simulink model "TestingModel"  (R2023b)
settings: Solver=VariableStepAuto  StartTime=0.0  StopTime=3.5  RelTol=1e-3
InitFcn:
  | run('Parameter_2M_DFIG_RSC.m')
values from neighbouring files (symbols this model uses):
  D = 0    [DefaultSimscapeValues.m]    (also in Newabccoordparam.m = 0.001)
  f = 60    [DefaultSimscapeValues.m]    (also in Newabccoordparam.m = 50)
  Fs = Vs*sqrt(2/3)/(2*pi*f)    [DefaultSimscapeValues.m]    (also in Newabccoordparam.m)
  fsw = 4e3    (= 4000)    [Newabccoordparam.m]
  J = 1.662    [DefaultSimscapeValues.m]    (also in Newabccoordparam.m = 127)
  ki_id = (wni^2)*Lr*sigma    (= 491.599501999)    [Newabccoordparam.m]
  ki_iq = ki_id    (= 491.599501999)    [Newabccoordparam.m]
  ki_n = ((wnn^2)*J)/p    (= 25400)    [Newabccoordparam.m]
  kp_id = (2*wni*sigma*Lr)-Rr    (= 0.5771)    [Newabccoordparam.m]
  kp_iq = kp_id    (= 0.5771)    [Newabccoordparam.m]
  kp_n = (2*wnn*J)/p    (= 2540)    [Newabccoordparam.m]
  Lm = 13.08/377    (= 0.0346949602122)    [DefaultSimscapeValues.m]    (also in Newabccoordparam.m = 0.0025)
  Lr = Lm + Lsi    (= 0.0354960212202)    [DefaultSimscapeValues.m]    (also in Newabccoordparam.m = 0.002587)
  Ls = Lm + Lsi    (= 0.0354960212202)    [DefaultSimscapeValues.m]    (also in Newabccoordparam.m = 0.002587)
  Lsi = 0.302/377    (= 0.000801061007958)    [DefaultSimscapeValues.m]    (also in Newabccoordparam.m = 8.7e-05)
  p = 2    [DefaultSimscapeValues.m]    (also in Newabccoordparam.m)
  Ps = 37300    [DefaultSimscapeValues.m]    (also in Newabccoordparam.m = 2000000)
  Rr = 0.228    [DefaultSimscapeValues.m]    (also in Newabccoordparam.m = 0.0029)
  Rs = 0.087    [DefaultSimscapeValues.m]    (also in Newabccoordparam.m = 0.0026)
  sigma = 1- Lm^2/(Ls*Lr)    (= 0.0446259584738)    [DefaultSimscapeValues.m]    (also in Newabccoordparam.m = 0.0661284179513)
  Tem = 12732    [Newabccoordparam.m]
  Vbus = Vr_stator*sqrt(2)    [Newabccoordparam.m]
  Vs = 460    [DefaultSimscapeValues.m]    (also in Newabccoordparam.m = 690)
undefined symbols (not defined in the file or in its folder): DiscIntNeverNeededParam
libraries: spsabctodq0Lib x3, eeGeneralControl x2, spsThreePhaseVIMeasurementLib x2, spsdq0toabcLib x2, spsAsynchronousMachineSIUnitsLib x1, spsDCVoltageSourceLib x1, spsGroundLib x1, spsPWMGenerator2LevelLib x1, spsThreePhaseProgrammableVoltageSourceLib x1, spsUniversalBridgeLib x1, sps_lib x1
settings Model: Creator=collins  LastModifiedBy=collins

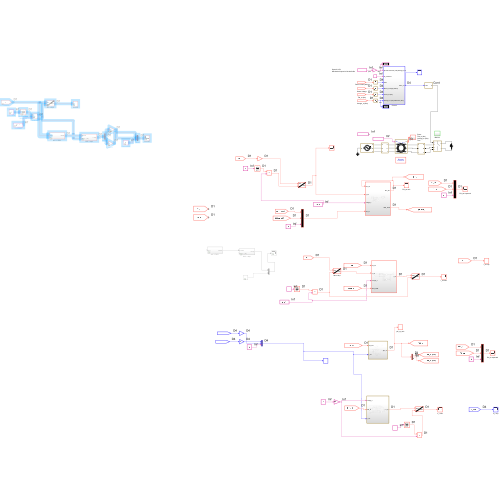
[thumbnail: Simulink's stored preview of the top-level diagram]
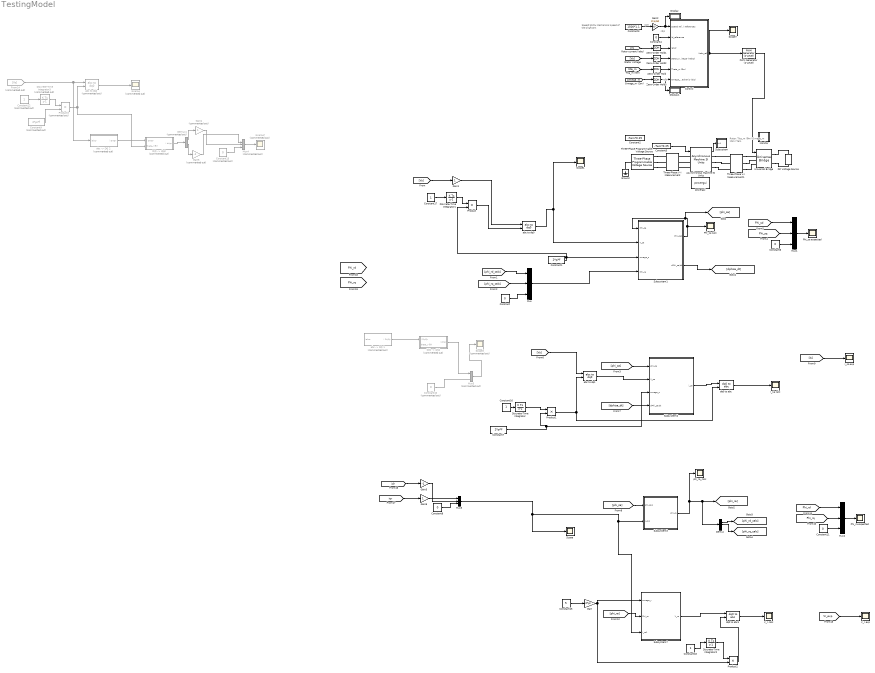
== system TestingModel ==
  note: rpm
  note: Rotor:
      | Tita_m (θm)
      | Omega_m (Ωm)
      | Tem
  note: rd/s
  note: rd/s
  note: Speed*110%
      | Mechanical speed of the shaft Ωm
  Asynchronous Machine SI Units : spsAsynchronousMachineSIUnitsLib/Asynchronous Machine SI Units  RotorType=Wound  PresetModel=No  MechanicalLoad=Torque Tm  ShowDetailedParameters=on  ReferenceFrame=Synchronous  Units=SI  MeasurementBus=off  NominalParameters=[ Ps Vs f ]  VoltageRatio=1  Stator=[ Rs , Lsi]  Rotor=[ Rr , Lsi]  Cage1=[ 0.022 0.226/377]  Cage2=[ 0.022 0.226/377]  Lm=Lm  Mechanical=[ J D 2 ]  PolePairs=2  InitialConditions=[1 0 0 0 0 0 0 0]  SimulateSaturation=off  Saturation=[14.03593122, 27.81365428, 53.79336849, 72.68890987, 97.98006896, 148.6815601, 215.7428561, 302.9841135, 420.4778367 ; 230, 322, 414, 460, 506, 552, 598, 644, 690]  LoadFlowParameters=1492000  TsPowergui=0  TsBlock=-1  IterativeModel=Trapezoidal non iterative  IterativeDiscreteModel=Trapezoidal non iterative  Pmec=0
      settings: AttributesFormatString=\n
  Constant{,4,6,8,11} (5 alike) : Constant  Value=0
  Constant1 : Constant  Value=2*pi*f
  Constant10 : Constant  Commented=on  Value=0
  Constant12 : Constant  Commented=on
  Constant13 : Constant  Commented=on  Value=0
  Constant15 : Constant  Value=5
  Constant16 : Constant
  Constant17 : Constant
  Constant18 : Constant
  Constant2 : Constant  Value=-Tem*0.25
  Constant3 : Constant  Value=1500*1.1
  Constant5 : Constant  Value=-Tem*0.25
  Constant7 : Constant  Value=2*pi*f
  Constant9 : Constant  Commented=on  Value=2*pi*f
  Control : Subsystem
  "D/Q -> d/q1" : Subsystem  Commented=on
  "D/Q -> d/q2" : Subsystem  Commented=on
  DC Voltage Source : spsDCVoltageSourceLib/DC Voltage Source  Amplitude=Vbus  Measurements=None
  Demux : Demux  Outputs=3
  Demux1 : Demux  Commented=on  Outputs=2
  Discrete-Time Integrator : DiscreteIntegrator  SampleTime=-1  ICPrevOutput=DiscIntNeverNeededParam  ICPrevScaledInput=DiscIntNeverNeededParam
  Discrete-Time Integrator1 : DiscreteIntegrator  SampleTime=-1  ICPrevOutput=DiscIntNeverNeededParam  ICPrevScaledInput=DiscIntNeverNeededParam
  Discrete-Time Integrator2 : DiscreteIntegrator  SampleTime=-1  ICPrevOutput=DiscIntNeverNeededParam  ICPrevScaledInput=DiscIntNeverNeededParam
  Discrete-Time Integrator3 : DiscreteIntegrator  Commented=on  SampleTime=-1  ICPrevOutput=DiscIntNeverNeededParam  ICPrevScaledInput=DiscIntNeverNeededParam
  Display : Display
  Display1 : Display
  From14 : From  Commented=on  GotoTag=Vs  TagVisibility=global
  Gain : Gain  Gain=2*pi
  Gain1 : Gain
  Gain2 : Gain  Gain=2*pi/60
  Gain3 : Gain  Gain=-1
  Gain4 : Gain  Commented=on
  Gain5 : Gain  Commented=on  Gain=-1
  Gain6 : Gain
  Ground : spsGroundLib/Ground  LConnTagsString=a
  Monitor : Subsystem
  Mux{,1..3} (4 alike) : Mux  Inputs=3
  Mux4 : Mux  Commented=on  Inputs=3
  Mux5 : Mux  Commented=on  Inputs=2
  PWM Generator (2-Level) : spsPWMGenerator2LevelLib/PWM Generator (2-Level)  ModulatorType=Three-phase bridge (6 pulses)  ModulatorMode=Unsynchronized  Fc=fsw  Pc=90  nF=27  MinMax="[ -1  1 ]"  SamplingTechnique=Natural  ModulatingSignals=off  m=0.8  Freq=60  Phase=0  Ts=0  ShowCarrierOutport=off
  Phi_ra expected : Scope
  Phi_sa calc : Scope
  Phi_sa expected : Scope
  Product : Product
  Product1 : Product
  Product2 : Product
  Product3 : Product  Commented=on
  Scope : Scope
  Scope1 : Scope
  Scope3 : Scope  Commented=on
  Scope7 : Scope
  Subsystem : Subsystem
  Subsystem1 : Subsystem
  Subsystem2 : Subsystem
  Subsystem3 : Subsystem
  Subsystem7 : Subsystem
  Three-Phase Programmable Voltage Source : spsThreePhaseProgrammableVoltageSourceLib/Three-Phase Programmable Voltage Source  PositiveSequence="[Vs  0 f]"  VariationEntity=None  VariationType=Table of time-amplitude pairs  VariationTypeAlt=Step  VariationStep=0.5  VariationRate=10  VariationMagnitude=0.3  VariationFrequency=2  VariationTiming=[1 2]  VariationPhaseA=off  Amplitudes=[1 0.8 1.2 1.0]  TimeValues=[0 0.1 0.15 0.2]  HarmonicGeneration=off  HarmonicA=[3 0.2 -25 0]  HarmonicB=[2 0.15 35 2]  Timing="[0.05  3]"  BusType=swing  Pref=0  Qref=0  Qmin=-inf  Qmax=inf
  Three-Phase V-I Measurement : spsThreePhaseVIMeasurementLib/Three-Phase V-I Measurement  VoltageMeasurement=phase-to-ground  SetLabelV=on  LabelV=Vs  Vpu=off  VpuLL=off  CurrentMeasurement=yes  SetLabelI=on  LabelI=Is  Ipu=off  Pbase=100e6  Vbase=500e3  OutputType=Complex  PhasorSimulation=off  PSBequivalent=0
  Three-Phase V-I Measurement1 : spsThreePhaseVIMeasurementLib/Three-Phase V-I Measurement  VoltageMeasurement=phase-to-phase  SetLabelV=on  LabelV=Vr  Vpu=off  VpuLL=off  CurrentMeasurement=yes  SetLabelI=on  LabelI=Ir  Ipu=off  Pbase=100e6  Vbase=500e3  OutputType=Complex  PhasorSimulation=off  PSBequivalent=0
  Universal Bridge : spsUniversalBridgeLib/Universal Bridge  Arms=3  SnubberResistance=1e5  SnubberCapacitance=inf  Device=Ideal Switches  Ron=1e-3  Lon=0  ForwardVoltages="[  0  0  ]"  ForwardVoltage=0  GTOparameters=[ 10e-6 , 20e-6 ]  IGBTparameters=[ 1e-6 , 2e-6 ]  Measurements=None  Measurements_2=None  converterType=Rectifier
  V_r calc : Scope
  V_r exp : Scope
  Zero-Order Hold{,1..3} (4 alike) : ZeroOrderHold  SampleTime=1/fsw
  "abc -> DQ 1" : Subsystem  Commented=on
  "abc -> DQ 2" : Subsystem  Commented=on
  abc to dq0 : spsabctodq0Lib/abc to dq0  Alignment=90 degrees behind phase A axis
  abc to dq1 : spsabctodq0Lib/abc to dq0  Alignment=90 degrees behind phase A axis
  abc to dq2 : spsabctodq0Lib/abc to dq0  Commented=on  Alignment=90 degrees behind phase A axis
  dq0 to abc : spsdq0toabcLib/dq0 to abc  Alignment=90 degrees behind phase A axis
  dq0 to abc1 : spsdq0toabcLib/dq0 to abc  Alignment=Aligned with phase A axis
  i_sa calc : Scope
  i_sa exp : Scope
  issame : Scope  Commented=on
  issame? : Scope  Commented=on
  phi_ra_calc : Scope
  powergui : sps_lib/powergui  Priority=1  SimulationMode=Discrete  SampleTime=15e-6  frequency=60  Iterations=50  frequencyindice=50  Pbase=100e6  ErrMax=1e-4  UnitsV=kV  UnitsW=MW  buscounter=0  FunctionMessages=off  echomessages=off  EnableUseOfTLC=off  CurrentSourceSwitches=off  DisableSnubberDevices=off  DisableRonSwitches=off  DisableVfSwitches=off  DisplayEquations=off  AutomaticDiscreteSolvers=off  SolverType=Tustin  Interpol=off  ExternalGateDelay=off  methode=off  Ts=0  x0status=blocks  SPID=off  SwTol=0  HookPort=off  NonlinearTolerance=1e-4  nMaxIteration=100  ContinueOnMaxIteration=off  RestoreLinks=warning  ResistiveCurrentMeasurement=off  Frange=[0:2:500]  Ylog=off  Xlog=on  ShowGrid=off  save=off  variable=ZData  structure=0  ZoomFFT=off  StartTime=0.0  cycles=1  DisplayStyle=1  fundamental=60  FreqAxis=off  MaxFrequency=1000  frequencyindicesteady=1  RmsSteady=1  display=off
  wires:
  Zero-Order Hold1/1 -> Control/3(iabcr)
  [Ir] -> Zero-Order Hold1/1
  [Vs] -> Zero-Order Hold2/1
  [omega_m] -> Zero-Order Hold3/1
  Zero-Order Hold2/1 -> Control/4(Stator_Voltage (Vabcs))
  Constant3/1 -> Gain2/1
  Zero-Order Hold/1 -> Control/5(Theta_m (θm))
  Constant4/1 -> Control/2(id_reference)
  Constant5/1 -> Asynchronous Machine SI Units/1
  PWM Generator (2-Level)/1 -> Universal Bridge/1
  Asynchronous Machine SI Units/1 -> Subsystem/1(In1)
  Zero-Order Hold3/1 -> Display1/1, Control/6(Omega_m (Ωm) Mechanic (rd/s))
  Gain2/1 -> Display/1, Control/1(Speed reference (rd/s) Omega_m (Ωm) references)
  [tita_m] -> Zero-Order Hold/1
  Control/1(Vabc_ref) -> Scope7/1, PWM Generator (2-Level)/1
  Subsystem1/1(Phi_sa1) -> Phi_sa calc/1, [phi_sa], Subsystem1/1(Phi_sa)
  Mux/1 -> Subsystem1/4(Phi_ra)
  Constant/1 -> Mux/3
  Constant1/1 -> Subsystem1/3(omega_s), Product/2
  Mux1/1 -> Phi_sa expected/1
  Constant6/1 -> Mux1/3
  [Phi_sq] -> Mux1/2
  [Phi_sd] -> Mux1/1
  [Vs] -> Gain1/1
  [phi_sa] -> Subsystem2/1(phi_sa)
  Constant7/1 -> Subsystem2/3(omega_s), Product1/2
  Subsystem1/2(dPhi_sa/dt) -> [dphisa_dt]
  [dphisa_dt] -> Subsystem2/4(dPhi_sa/dt)
  [Is] -> i_sa exp/1
  Subsystem2/1(i_sa) -> dq0 to abc/1
  dq0 to abc/1 -> i_sa calc/1
  Subsystem3/1(phi_ra) -> Demux/1, [phi_ra], phi_ra_calc/1
  Constant11/1 -> Mux2/3
  Mux2/1 -> Phi_ra expected/1
  [Phi_rq] -> Mux2/2
  [Phi_rd] -> Mux2/1
  Demux/1 -> [phi_rd_calc]
  Demux/2 -> [phi_rq_calc]
  [phi_ra] -> Subsystem7/2(Phi_ra)
  dq0 to abc1/1 -> V_r calc/1
  [Vr_exp] -> V_r exp/1
  Product2/1 -> dq0 to abc1/2
  Constant8/1 -> Mux3/3
  Gain/1 -> Subsystem7/1(omega_r), Product2/2
  Subsystem7/1(V_ra) -> dq0 to abc1/1
  Mux3/1 -> Subsystem7/3(i_ra1), Subsystem3/2(i_ra1), Scope/1
  Product/1 -> abc to dq0/2
  [phi_sa] -> Subsystem3/1(phi_sa1)
  Constant15/1 -> Gain/1
  Discrete-Time Integrator/1 -> Product1/1
  Constant16/1 -> Discrete-Time Integrator/1
  Discrete-Time Integrator1/1 -> Product/1
  Constant17/1 -> Discrete-Time Integrator1/1
  Discrete-Time Integrator2/1 -> Product2/1
  Constant18/1 -> Discrete-Time Integrator2/1
  abc to dq0/1 -> Scope1/1, Subsystem1/2(V_sa)
  Gain1/1 -> abc to dq0/1
  [phi_rd_calc] -> Mux/1
  [phi_rq_calc] -> Mux/2
  [Vs] -> abc to dq1/1
  Mux5/1 -> Scope3/1
  "abc -> DQ 1"/1(i Dr/Qr) -> "D/Q -> d/q1"/1(i Dr/Qr)
  "D/Q -> d/q1"/1(i dr/qr) -> Mux5/1
  Product1/1 -> abc to dq1/2, dq0 to abc/2
  Constant10/1 -> ?
  abc to dq1/1 -> Subsystem2/2(V_sa)
  From14/1 -> "abc -> DQ 2"/1(iabcr), abc to dq2/1
  "abc -> DQ 2"/1(i Dr/Qr) -> "D/Q -> d/q2"/1(i Dr/Qr)
  [idr] -> Gain3/1
  Gain3/1 -> Mux3/2
  [iqr] -> Gain6/1
  Discrete-Time Integrator3/1 -> Product3/1
  Constant9/1 -> Product3/2
  Constant12/1 -> Discrete-Time Integrator3/1
  abc to dq2/1 -> issame/1
  Product3/1 -> abc to dq2/2, "D/Q -> d/q2"/2(theta_r (θr))
  "D/Q -> d/q2"/1(i dr/qr) -> Demux1/1
  Demux1/2 -> Gain5/1
  Demux1/1 -> Gain4/1
  Constant13/1 -> Mux4/3
  Mux4/1 -> issame?/1
  Gain4/1 -> Mux4/2
  Gain5/1 -> Mux4/1
  Gain6/1 -> Mux3/1
  connections:
  Three-Phase V-I Measurement1/LConn2 -- Universal Bridge/LConn2
  Asynchronous Machine SI Units/LConn1 -- Three-Phase V-I Measurement/RConn1
  Universal Bridge/RConn1 -- DC Voltage Source/RConn1
  Asynchronous Machine SI Units/LConn2 -- Three-Phase V-I Measurement/RConn2
  Asynchronous Machine SI Units/RConn1 -- Three-Phase V-I Measurement1/RConn1
  Asynchronous Machine SI Units/LConn3 -- Three-Phase V-I Measurement/RConn3
  Asynchronous Machine SI Units/RConn3 -- Three-Phase V-I Measurement1/RConn3
  Three-Phase Programmable Voltage Source/LConn1 -- Ground/LConn1
  Three-Phase Programmable Voltage Source/RConn1 -- Three-Phase V-I Measurement/LConn1
  Three-Phase V-I Measurement1/LConn1 -- Universal Bridge/LConn1
  Asynchronous Machine SI Units/RConn2 -- Three-Phase V-I Measurement1/RConn2
  Three-Phase Programmable Voltage Source/RConn3 -- Three-Phase V-I Measurement/LConn3
  Three-Phase V-I Measurement1/LConn3 -- Universal Bridge/LConn3
  Universal Bridge/RConn2 -- DC Voltage Source/LConn1
  Three-Phase Programmable Voltage Source/RConn2 -- Three-Phase V-I Measurement/LConn2

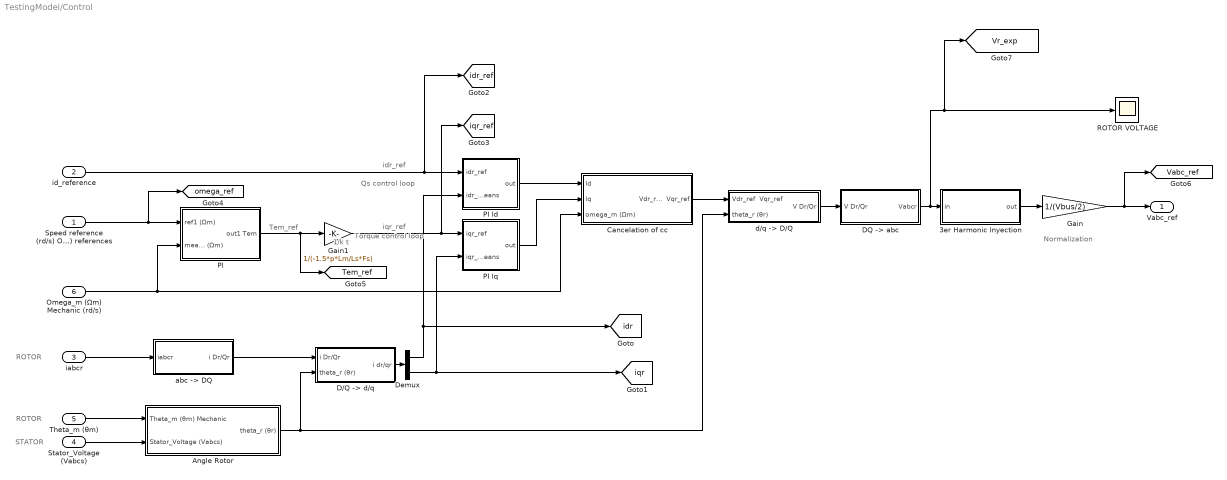
== system TestingModel/Control ==
  note: Normalization
  note: Torque control loop
  note: 1/k t
  note: STATOR
  note: ROTOR
  note: iqr_ref
  note: Tem_ref
  note: idr_ref
  note: ROTOR
  note: Qs control loop
  Speed reference (rd/s) Omega_m (Ωm) references : Inport
  id_reference : Inport  Port=2
  iabcr : Inport  Port=3
  Stator_Voltage (Vabcs) : Inport  Port=4
  Theta_m (θm) : Inport  Port=5
  Omega_m (Ωm) Mechanic (rd/s) : Inport  Port=6
  " Angle Rotor" : Subsystem
  3er Harmonic Inyection : Subsystem
  Cancelation of cc : Subsystem
  "D/Q -> d/q" : Subsystem
  "DQ -> abc" : Subsystem
  Demux : Demux  Outputs=2
  Gain : Gain  Gain=1/(Vbus/2)
  Gain1 : Gain  Gain=1/(-1.5*p*Lm/Ls*Fs)
  PI : Subsystem
  PI Id : Subsystem
  PI Iq : Subsystem
  ROTOR VOLTAGE : Scope
  "abc -> DQ " : Subsystem
  "d/q -> D/Q " : Subsystem
  Vabc_ref : Outport  VectorParamsAs1DForOutWhenUnconnected=off
  tag scope: Tem_ref=global, Vabc_ref=global, Vr_exp=global, idr=global, idr_ref=global, iqr=global, iqr_ref=global, omega_ref=global
  wires:
  "DQ -> abc"/1(Vabcr) -> [Vr_exp], ROTOR VOLTAGE/1, 3er Harmonic Inyection/1(in)
  "d/q -> D/Q "/1(V Dr/Qr) -> "DQ -> abc"/1(V Dr/Qr)
  iabcr/1 -> "abc -> DQ "/1(iabcr)
  "abc -> DQ "/1(i Dr/Qr) -> "D/Q -> d/q"/1(i Dr/Qr)
  3er Harmonic Inyection/1(out) -> Gain/1
  Theta_m (θm)/1 -> " Angle Rotor"/1(Theta_m (θm) Mechanic)
  Stator_Voltage (Vabcs)/1 -> " Angle Rotor"/2(Stator_Voltage (Vabcs))
  " Angle Rotor"/1(theta_r (θr)) -> "D/Q -> d/q"/2(theta_r (θr)), "d/q -> D/Q "/2(theta_r (θr))
  PI Id/1(out) -> Cancelation of cc/1(Id)
  PI Iq/1(out) -> Cancelation of cc/2(Iq)
  Omega_m (Ωm) Mechanic (rd/s)/1 -> PI/2("means1 (Ωm) "), Cancelation of cc/3(omega_m (Ωm))
  "D/Q -> d/q"/1(i dr/qr) -> Demux/1
  Demux/2 -> PI Iq/2(iqr_means), [iqr]
  Demux/1 -> PI Id/2(idr_means), [idr]
  PI/1(out1 Tem) -> [Tem_ref], Gain1/1
  Gain1/1 -> [iqr_ref], PI Iq/1(iqr_ref)
  id_reference/1 -> [idr_ref], PI Id/1(idr_ref)
  Cancelation of cc/1(Vdr_ref  Vqr_ref) -> "d/q -> D/Q "/1(Vdr_ref  Vqr_ref)
  Speed reference (rd/s) Omega_m (Ωm) references/1 -> [omega_ref], PI/1("ref1 (Ωm) ")
  Gain/1 -> [Vabc_ref], Vabc_ref/1

== system TestingModel/D//Q -> d//q1 ==
  i Dr/Qr : Inport
  theta_r (θr) : Inport  Port=2
  Fcn : Fcn  Expr=u[1]*cos(u[3])+u[2]*sin(u[3])
  Fcn1 : Fcn  Expr=-u[1]*sin(u[3])+u[2]*cos(u[3])
  Mux : Mux  Inputs=2
  Mux1 : Mux  Inputs=2
  i dr/qr : Outport  VectorParamsAs1DForOutWhenUnconnected=off
  wires:
  Mux/1 -> i dr/qr/1
  Fcn/1 -> Mux/1
  Fcn1/1 -> Mux/2
  i Dr/Qr/1 -> Mux1/1
  Mux1/1 -> Fcn1/1, Fcn/1
  theta_r (θr)/1 -> Mux1/2

== system TestingModel/D//Q -> d//q2 ==
  i Dr/Qr : Inport
  theta_r (θr) : Inport  Port=2
  Fcn : Fcn  Expr=u[1]*cos(u[3])+u[2]*sin(u[3])
  Fcn1 : Fcn  Expr=-u[1]*sin(u[3])+u[2]*cos(u[3])
  Mux : Mux  Inputs=2
  Mux1 : Mux  Inputs=2
  i dr/qr : Outport  VectorParamsAs1DForOutWhenUnconnected=off
  wires:
  Mux/1 -> i dr/qr/1
  Fcn/1 -> Mux/1
  Fcn1/1 -> Mux/2
  i Dr/Qr/1 -> Mux1/1
  Mux1/1 -> Fcn1/1, Fcn/1
  theta_r (θr)/1 -> Mux1/2

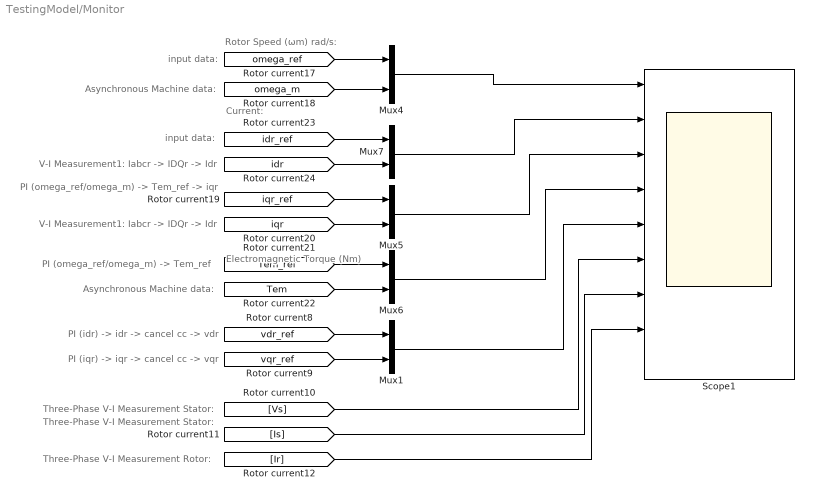
== system TestingModel/Monitor ==
  note: Electromagnetic Torque (Nm)
  note: Three-Phase V-I Measurement Stator:
  note: PI (idr) -> idr -> cancel cc -> vdr
  note: PI (omega_ref/omega_m) -> Tem_ref -> iqr
  note: V-I Measurement1: Iabcr -> IDQr -> Idr
  note: input data:
  note: Current:
  note: Rotor Speed (ωm) rad/s:
  note: Asynchronous Machine data:
  note: input data:
  note: V-I Measurement1: Iabcr -> IDQr -> Idr
  note: PI (omega_ref/omega_m) -> Tem_ref
  note: Asynchronous Machine data:
  note: PI (iqr) -> iqr -> cancel cc -> vqr
  note: Three-Phase V-I Measurement Stator:
  note: Three-Phase V-I Measurement Rotor:
  Mux{1,4..7} (5 alike) : Mux  Inputs=2
  Scope1 : Scope  NumInputPorts=9
  wires:
  [omega_m] -> Mux4/2
  [omega_ref] -> Mux4/1
  [iqr_ref] -> Mux5/1
  [iqr] -> Mux5/2
  [Tem_ref] -> Mux6/1
  [idr] -> Mux7/2
  [idr_ref] -> Mux7/1
  Mux4/1 -> Scope1/1
  [vdr_ref] -> Mux1/1
  [vqr_ref] -> Mux1/2
  Mux7/1 -> Scope1/2
  Mux5/1 -> Scope1/3
  Mux6/1 -> Scope1/4
  Mux1/1 -> Scope1/5
  [Vs] -> Scope1/6
  [Is] -> Scope1/7
  [Ir] -> Scope1/8
  [Tem] -> Mux6/2

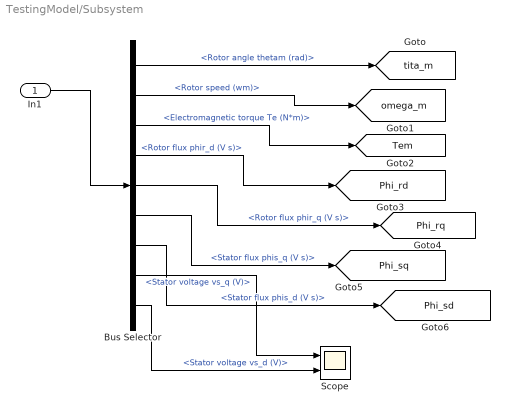
== system TestingModel/Subsystem ==
  In1 : Inport
  Bus Selector : BusSelector  OutputSignals=Mechanical.Rotor angle thetam (rad),Mechanical.Rotor speed (wm),Mechanical.Electromagnetic torque Te (N*m),Rotor measurements.Rotor flux phir_d (V s),Rotor measurements.Rotor flux phir_q (V s),Stator measurements.Stator flux phis_q (V s),Stator measurements.Stator flux phis_d (V s),Stator measurements.Stator voltage vs_q (V),Stator measurements.Stator voltage vs_d (V)
  Scope : Scope  NumInputPorts=2
  tag scope: Phi_rd=global, Phi_rq=global, Phi_sd=global, Phi_sq=global, Tem=global, omega_m=global, tita_m=global
  wires:
  Bus Selector/2 -> [omega_m]  "<Rotor speed (wm)>"
  In1/1 -> Bus Selector/1
  Bus Selector/1 -> [tita_m]  "<Rotor angle thetam (rad)>"
  Bus Selector/3 -> [Tem]  "<Electromagnetic torque Te (N*m)>"
  Bus Selector/4 -> [Phi_rd]  "<Rotor flux phir_d (V s)>"
  Bus Selector/5 -> [Phi_rq]  "<Rotor flux phir_q (V s)>"
  Bus Selector/6 -> [Phi_sq]  "<Stator flux phis_q (V s)>"
  Bus Selector/7 -> [Phi_sd]  "<Stator flux phis_d (V s)>"
  Bus Selector/8 -> Scope/1  "<Stator voltage vs_q (V)>"
  Bus Selector/9 -> Scope/2  "<Stator voltage vs_d (V)>"

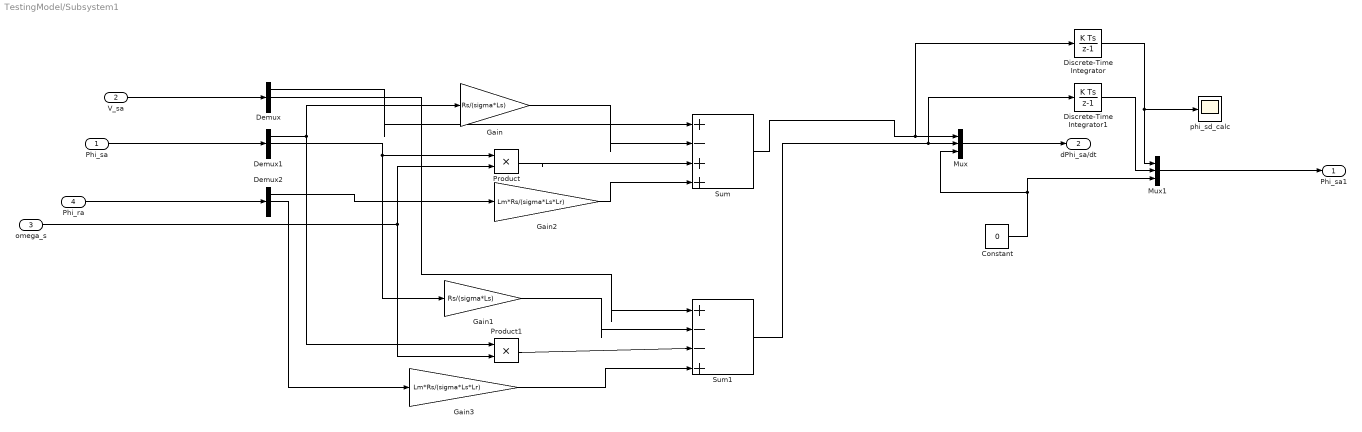
== system TestingModel/Subsystem1 ==
  Phi_sa : Inport
  V_sa : Inport  Port=2
  omega_s : Inport  Port=3
  Phi_ra : Inport  Port=4
  Constant : Constant  Value=0
  Demux : Demux  Outputs=3
  Demux1 : Demux  Outputs=3
  Demux2 : Demux  Outputs=3
  Discrete-Time Integrator : DiscreteIntegrator  SampleTime=-1  ICPrevOutput=DiscIntNeverNeededParam  ICPrevScaledInput=DiscIntNeverNeededParam
  Discrete-Time Integrator1 : DiscreteIntegrator  SampleTime=-1  ICPrevOutput=DiscIntNeverNeededParam  ICPrevScaledInput=DiscIntNeverNeededParam
  Gain : Gain  Gain=Rs/(sigma*Ls)
  Gain1 : Gain  Gain=Rs/(sigma*Ls)
  Gain2 : Gain  Gain=Lm*Rs/(sigma*Ls*Lr)
  Gain3 : Gain  Gain=Lm*Rs/(sigma*Ls*Lr)
  Mux : Mux  Inputs=3
  Mux1 : Mux  Inputs=3
  Product : Product
  Product1 : Product
  Sum : Sum  Inputs=|+-++
  Sum1 : Sum  Inputs=|+--+
  phi_sd_calc : Scope
  Phi_sa1 : Outport
  dPhi_sa/dt : Outport  Port=2
  wires:
  Gain/1 -> Sum/2
  Gain2/1 -> Sum/4
  Product/1 -> Sum/3
  Mux/1 -> dPhi_sa/dt/1
  Demux/1 -> Sum/1
  Gain1/1 -> Sum1/2
  Gain3/1 -> Sum1/4
  Product1/1 -> Sum1/3
  Demux/2 -> Sum1/1
  Mux1/1 -> Phi_sa1/1
  Demux1/1 -> Product1/1, Gain/1
  Demux2/1 -> Gain2/1
  Demux1/2 -> Product/1, Gain1/1
  Demux2/2 -> Gain3/1
  Constant/1 -> Mux1/3, Mux/3
  Discrete-Time Integrator/1 -> Mux1/1, phi_sd_calc/1
  Discrete-Time Integrator1/1 -> Mux1/2
  Phi_sa/1 -> Demux1/1
  Phi_ra/1 -> Demux2/1
  omega_s/1 -> Product/2, Product1/2
  Sum/1 -> Discrete-Time Integrator/1, Mux/1
  Sum1/1 -> Discrete-Time Integrator1/1, Mux/2
  V_sa/1 -> Demux/1

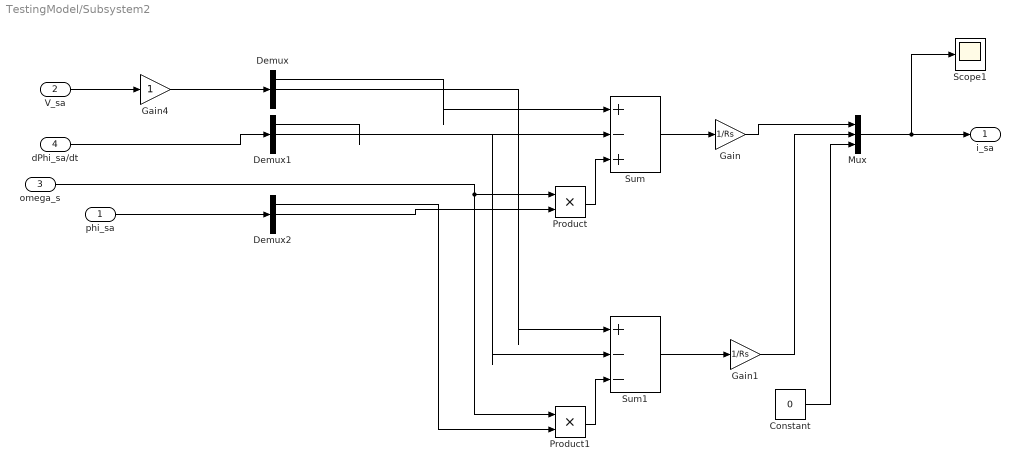
== system TestingModel/Subsystem2 ==
  phi_sa : Inport
  V_sa : Inport  Port=2
  omega_s : Inport  Port=3
  dPhi_sa/dt : Inport  Port=4
  Constant : Constant  Value=0
  Demux : Demux  Outputs=3
  Demux1 : Demux  Outputs=3
  Demux2 : Demux  Outputs=3
  Gain : Gain  Gain=1/Rs
  Gain1 : Gain  Gain=1/Rs
  Gain4 : Gain
  Mux : Mux  Inputs=3
  Product : Product
  Product1 : Product
  Scope1 : Scope
  Sum : Sum  Inputs=|+-+
  Sum1 : Sum  Inputs=|+--
  i_sa : Outport
  wires:
  Product/1 -> Sum/3
  Constant/1 -> Mux/3
  Demux/1 -> Sum/1
  Demux1/1 -> Sum/2
  Demux2/2 -> Product/2
  Product1/1 -> Sum1/3
  Sum/1 -> Gain/1
  Sum1/1 -> Gain1/1
  Demux/2 -> Sum1/1
  Demux1/2 -> Sum1/2
  Demux2/1 -> Product1/2
  Gain/1 -> Mux/1
  Gain1/1 -> Mux/2
  Mux/1 -> Scope1/1, i_sa/1
  V_sa/1 -> Gain4/1
  dPhi_sa/dt/1 -> Demux1/1
  phi_sa/1 -> Demux2/1
  omega_s/1 -> Product1/1, Product/1
  Gain4/1 -> Demux/1

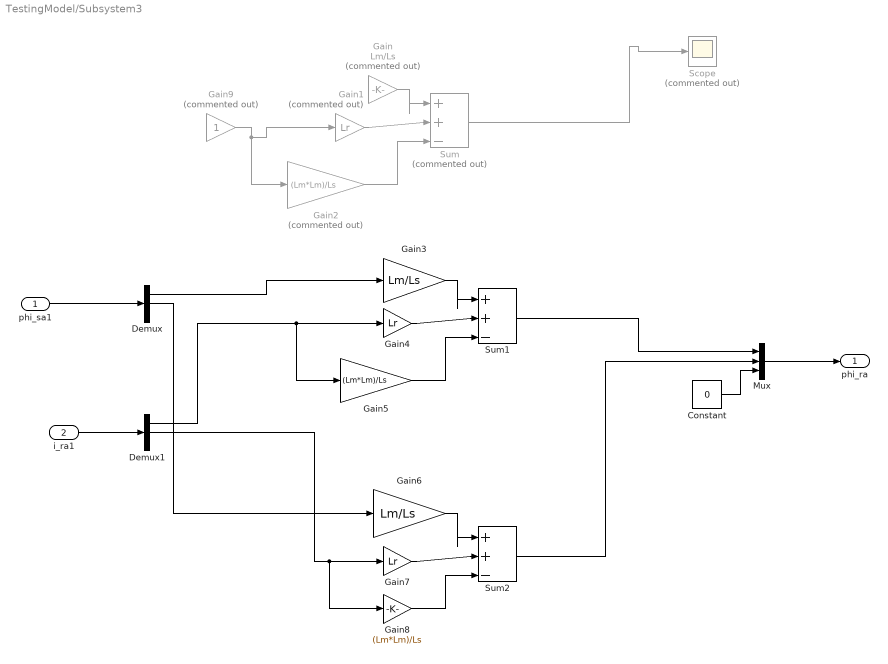
== system TestingModel/Subsystem3 ==
  phi_sa1 : Inport
  i_ra1 : Inport  Port=2
  Constant : Constant  Value=0
  Demux : Demux  Outputs=3
  Demux1 : Demux  Outputs=3
  Gain : Gain  Commented=on  Gain=Lm/Ls
  Gain1 : Gain  Commented=on  Gain=Lr
  Gain2 : Gain  Commented=on  Gain=(Lm*Lm)/Ls
  Gain3 : Gain  Gain=Lm/Ls
  Gain4 : Gain  Gain=Lr
  Gain5 : Gain  Gain=(Lm*Lm)/Ls
  Gain6 : Gain  Gain=Lm/Ls
  Gain7 : Gain  Gain=Lr
  Gain8 : Gain  Gain=(Lm*Lm)/Ls
  Gain9 : Gain  Commented=on
  Mux : Mux  Inputs=3
  Scope : Scope  Commented=on
  Sum : Sum  Commented=on  Inputs=|++-  RndMeth=Round
  Sum1 : Sum  Inputs=|++-  RndMeth=Round
  Sum2 : Sum  Inputs=|++-  RndMeth=Round
  phi_ra : Outport
  wires:
  Gain/1 -> Sum/1
  Gain1/1 -> Sum/2
  Gain2/1 -> Sum/3
  Sum/1 -> Scope/1
  Gain3/1 -> Sum1/1
  Gain5/1 -> Sum1/3
  Gain4/1 -> Sum1/2
  Gain6/1 -> Sum2/1
  Gain8/1 -> Sum2/3
  Gain7/1 -> Sum2/2
  Constant/1 -> Mux/3
  Sum1/1 -> Mux/1
  Sum2/1 -> Mux/2
  Gain9/1 -> Gain2/1, Gain1/1
  phi_sa1/1 -> Demux/1
  i_ra1/1 -> Demux1/1
  Mux/1 -> phi_ra/1
  Demux/1 -> Gain3/1
  Demux/2 -> Gain6/1
  Demux1/1 -> Gain5/1, Gain4/1
  Demux1/2 -> Gain8/1, Gain7/1

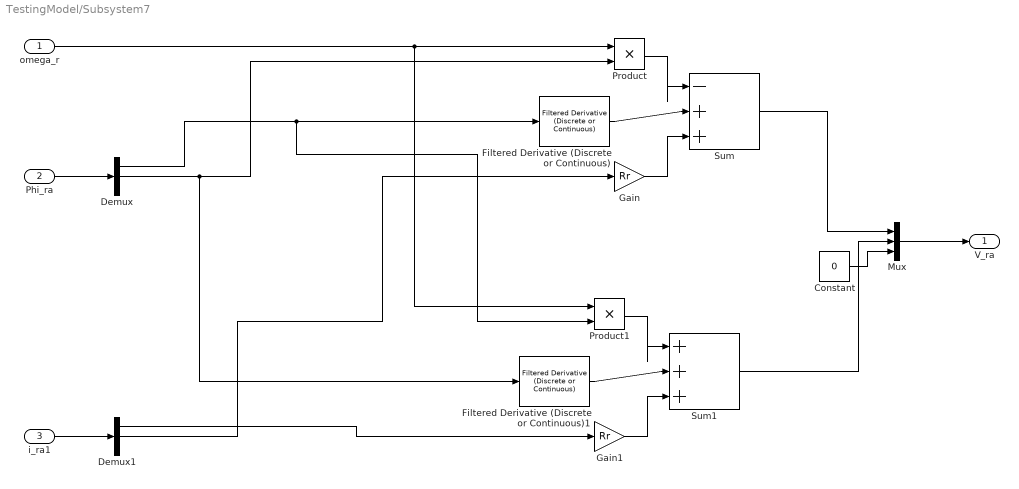
== system TestingModel/Subsystem7 ==
  omega_r : Inport
  Phi_ra : Inport  Port=2
  i_ra1 : Inport  Port=3
  Constant : Constant  Value=0
  Demux : Demux  Outputs=3
  Demux1 : Demux  Outputs=3
  Filtered Derivative (Discrete or Continuous) : eeGeneralControl/Filtered Derivative (Discrete or Continuous)  K=1  T=0.1  B=inf  A=-inf  minRatio=10  init_option=Inherited from block input  x0=0  Ts=-1
      settings: LibrarySourceBlock=|
      | ee_sl_lib/General Control/Filtered Derivative
      | (Discrete or Continuous)
  Filtered Derivative (Discrete or Continuous)1 : eeGeneralControl/Filtered Derivative (Discrete or Continuous)  K=1  T=0.1  B=inf  A=-inf  minRatio=10  init_option=Inherited from block input  x0=0  Ts=-1
      settings: LibrarySourceBlock=|
      | ee_sl_lib/General Control/Filtered Derivative
      | (Discrete or Continuous)
  Gain : Gain  Gain=Rr
  Gain1 : Gain  Gain=Rr
  Mux : Mux  Inputs=3
  Product : Product
  Product1 : Product
  Sum : Sum  Inputs=|-++
  Sum1 : Sum  Inputs=|+++
  V_ra : Outport
  wires:
  Product/1 -> Sum/1
  Gain/1 -> Sum/3
  Filtered Derivative (Discrete or Continuous)/1 -> Sum/2
  Gain1/1 -> Sum1/3
  Filtered Derivative (Discrete or Continuous)1/1 -> Sum1/2
  Product1/1 -> Sum1/1
  i_ra1/1 -> Demux1/1
  omega_r/1 -> Product1/1, Product/1
  Demux1/1 -> Gain1/1
  Demux1/2 -> Gain/1
  Phi_ra/1 -> Demux/1
  Demux/2 -> Filtered Derivative (Discrete or Continuous)1/1, Product/2
  Demux/1 -> Product1/2, Filtered Derivative (Discrete or Continuous)/1
  Constant/1 -> Mux/3
  Sum1/1 -> Mux/2
  Sum/1 -> Mux/1
  Mux/1 -> V_ra/1

== system TestingModel/abc -> DQ 1 ==
  note: iQr
  note: iDr
  iabcr : Inport
  Fcn : Fcn  Expr=2/3*(u[1]-u[2]/2-u[3]/2)
  Fcn1 : Fcn  Expr=2/3*(u[2]*(sqrt(3)/2)-u[3]*(sqrt(3)/2))
  Mux : Mux  Inputs=2
  i Dr/Qr : Outport  VectorParamsAs1DForOutWhenUnconnected=off
  wires:
  Mux/1 -> i Dr/Qr/1
  iabcr/1 -> Fcn1/1, Fcn/1
  Fcn/1 -> Mux/1
  Fcn1/1 -> Mux/2

== system TestingModel/abc -> DQ 2 ==
  note: iQr
  note: iDr
  iabcr : Inport
  Fcn : Fcn  Expr=2/3*(u[1]-u[2]/2-u[3]/2)
  Fcn1 : Fcn  Expr=2/3*(u[2]*(sqrt(3)/2)-u[3]*(sqrt(3)/2))
  Mux : Mux  Inputs=2
  i Dr/Qr : Outport  VectorParamsAs1DForOutWhenUnconnected=off
  wires:
  Mux/1 -> i Dr/Qr/1
  iabcr/1 -> Fcn1/1, Fcn/1
  Fcn/1 -> Mux/1
  Fcn1/1 -> Mux/2

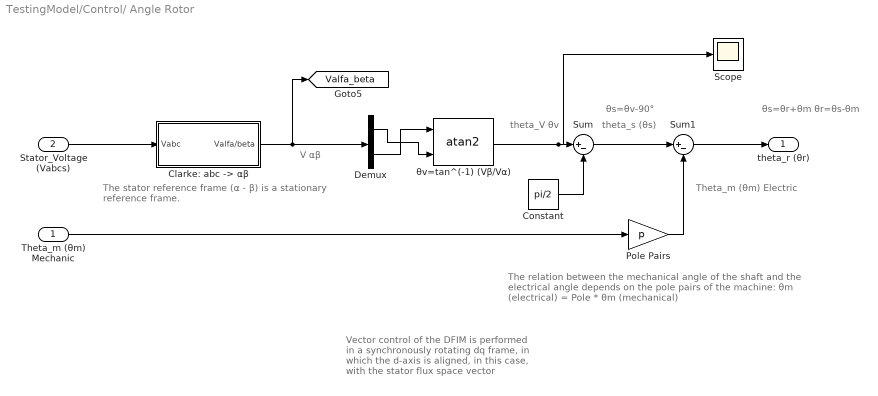
== system TestingModel/Control/ Angle Rotor ==
  note: Theta_m (θm)
      | Electric
  note: theta_V θv
  note: The stator reference frame (α - β) is a stationary
      | reference frame.
  note: The relation between the mechanical angle of the shaft and the
      | electrical angle depends on the pole pairs of the machine:
      |
      | θm (electrical) = Pole * θm (mechanical)
  note: theta_s (θs)
  note: V αβ
  note: θs=θv-90°
  note: θs=θr+θm
      | θr=θs-θm
  note: Vector control of the DFIM is performed in a synchronously rotating dq frame, in which the d-axis is aligned, in this case, with the stator flux space vector
  Theta_m (θm) Mechanic : Inport
  Stator_Voltage (Vabcs) : Inport  Port=2
  "Clarke: abc -> αβ " : Subsystem
  Constant : Constant  Value=pi/2
  Demux : Demux  Outputs=2
  Pole Pairs : Gain  Gain=p
  Scope : Scope
  Sum : Sum  Inputs=|+-
  Sum1 : Sum  Inputs=|+-
  θv=tan^(-1) (Vβ/Vα) : Trigonometry  Operator=atan2
  theta_r (θr) : Outport  VectorParamsAs1DForOutWhenUnconnected=off
  tag scope: Valfa_beta=global
  wires:
  Stator_Voltage (Vabcs)/1 -> "Clarke: abc -> αβ "/1(Vabc)
  Demux/2 -> θv=tan^(-1) (Vβ/Vα)/1
  Demux/1 -> θv=tan^(-1) (Vβ/Vα)/2
  "Clarke: abc -> αβ "/1("Valfa/beta ") -> Demux/1, [Valfa_beta]
  θv=tan^(-1) (Vβ/Vα)/1 -> Scope/1, Sum/1
  Constant/1 -> Sum/2
  Theta_m (θm) Mechanic/1 -> Pole Pairs/1
  Sum/1 -> Sum1/1
  Sum1/1 -> theta_r (θr)/1
  Pole Pairs/1 -> Sum1/2

== system TestingModel/Control/3er Harmonic Inyection ==
  in : Inport
  Gain : Gain  Gain=-0.5
  MinMax : MinMax
  MinMax1 : MinMax  Function=max
  Scope : Scope
  Sum : Sum  Inputs=|++
  Sum1 : Sum  Inputs=|++
  out : Outport  VectorParamsAs1DForOutWhenUnconnected=off
  wires:
  in/1 -> Sum1/1, MinMax1/1, MinMax/1
  MinMax/1 -> Sum/1
  MinMax1/1 -> Sum/2
  Sum1/1 -> out/1
  Sum/1 -> Gain/1
  Gain/1 -> Scope/1, Sum1/2

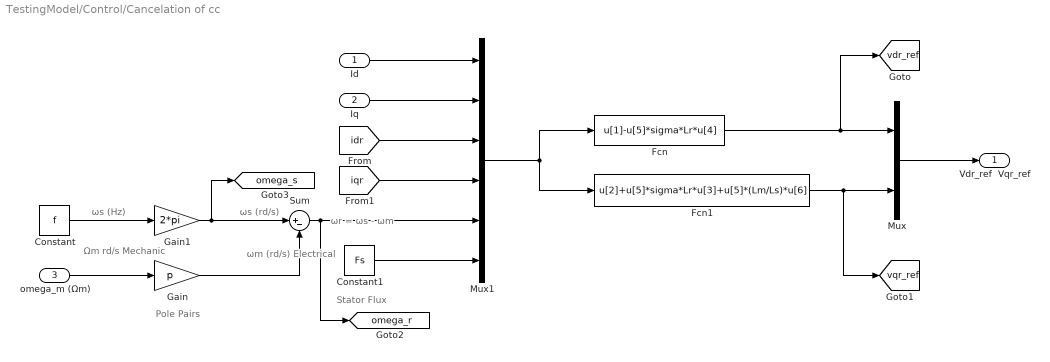
== system TestingModel/Control/Cancelation of cc ==
  note: Stator Flux
  note: Ωm rd/s
      | Mechanic
  note: ωs (Hz)
  note: Pole Pairs
  note: ωr = ωs - ωm
  note: ωs (rd/s)
  note: ωm (rd/s)
      | Electrical
  Id : Inport
  Iq : Inport  Port=2
  omega_m (Ωm) : Inport  Port=3
  Constant : Constant  Value=f
  Constant1 : Constant  Value=Fs
  Fcn : Fcn  Expr=u[1]-u[5]*sigma*Lr*u[4]
  Fcn1 : Fcn  Expr=u[2]+u[5]*sigma*Lr*u[3]+u[5]*(Lm/Ls)*u[6]
  Gain : Gain  Gain=p
  Gain1 : Gain  Gain=2*pi
  Mux : Mux  Inputs=2
  Mux1 : Mux  Inputs=6
  Sum : Sum  Inputs=|+-
  Vdr_ref  Vqr_ref : Outport  VectorParamsAs1DForOutWhenUnconnected=off
  tag scope: omega_r=global, omega_s=global, vdr_ref=global, vqr_ref=global
  wires:
  Mux/1 -> Vdr_ref  Vqr_ref/1
  Fcn/1 -> [vdr_ref], Mux/1
  Fcn1/1 -> [vqr_ref], Mux/2
  Id/1 -> Mux1/1
  Iq/1 -> Mux1/2
  Mux1/1 -> Fcn1/1, Fcn/1
  [idr] -> Mux1/3
  [iqr] -> Mux1/4
  Constant1/1 -> Mux1/6
  omega_m (Ωm)/1 -> Gain/1
  Gain/1 -> Sum/2
  Constant/1 -> Gain1/1
  Gain1/1 -> [omega_s], Sum/1
  Sum/1 -> [omega_r], Mux1/5

== system TestingModel/Control/D//Q -> d//q ==
  i Dr/Qr : Inport
  theta_r (θr) : Inport  Port=2
  Fcn : Fcn  Expr=u[1]*cos(u[3])+u[2]*sin(u[3])
  Fcn1 : Fcn  Expr=-u[1]*sin(u[3])+u[2]*cos(u[3])
  Mux : Mux  Inputs=2
  Mux1 : Mux  Inputs=2
  i dr/qr : Outport  VectorParamsAs1DForOutWhenUnconnected=off
  wires:
  Mux/1 -> i dr/qr/1
  Fcn/1 -> Mux/1
  Fcn1/1 -> Mux/2
  i Dr/Qr/1 -> Mux1/1
  Mux1/1 -> Fcn1/1, Fcn/1
  theta_r (θr)/1 -> Mux1/2

== system TestingModel/Control/DQ -> abc ==
  V Dr/Qr : Inport
  Fcn : Fcn  Expr=u(1)
  Fcn1 : Fcn  Expr=-(u[1]/2)+u[2]*(sqrt(3)/2)
  Fcn2 : Fcn  Expr=-(u[1]/2)-u[2]*(sqrt(3)/2)
  Mux : Mux  Inputs=3
  Vabcr : Outport  VectorParamsAs1DForOutWhenUnconnected=off
  wires:
  Mux/1 -> Vabcr/1
  V Dr/Qr/1 -> Fcn2/1, Fcn1/1, Fcn/1
  Fcn/1 -> Mux/1
  Fcn1/1 -> Mux/2
  Fcn2/1 -> Mux/3

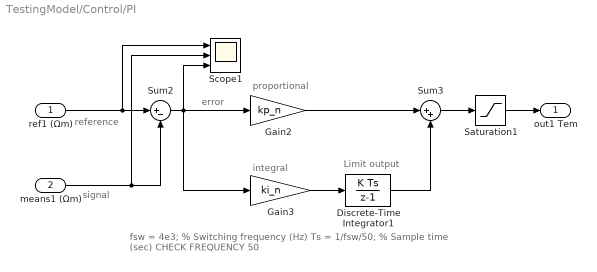
== system TestingModel/Control/PI ==
  note: Limit output
  note: proportional
  note: reference
  note: error
  note: fsw = 4e3;                  % Switching frequency (Hz)
      | Ts = 1/fsw/50;            % Sample time (sec) CHECK FREQUENCY 50
  note: signal
  note: integral
  "ref1 (Ωm) " : Inport
  "means1 (Ωm) " : Inport  Port=2
  Discrete-Time Integrator1 : DiscreteIntegrator  SampleTime=1/fsw  LimitOutput=on  UpperSaturationLimit=Tem  LowerSaturationLimit=-Tem  ICPrevOutput=DiscIntNeverNeededParam  ICPrevScaledInput=DiscIntNeverNeededParam
  Gain2 : Gain  Gain=kp_n
  Gain3 : Gain  Gain=ki_n
  Saturation1 : Saturate  UpperLimit=Tem  LowerLimit=-Tem
  Scope1 : Scope  NumInputPorts=3
  Sum2 : Sum  Inputs=|+-
  Sum3 : Sum  Inputs=|++
  out1 Tem : Outport  VectorParamsAs1DForOutWhenUnconnected=off
  wires:
  Gain2/1 -> Sum3/1
  Sum3/1 -> Saturation1/1
  "ref1 (Ωm) "/1 -> Scope1/1, Sum2/1
  "means1 (Ωm) "/1 -> Scope1/2, Sum2/2
  Sum2/1 -> Scope1/3, Gain3/1, Gain2/1
  Gain3/1 -> Discrete-Time Integrator1/1
  Discrete-Time Integrator1/1 -> Sum3/2
  Saturation1/1 -> out1 Tem/1

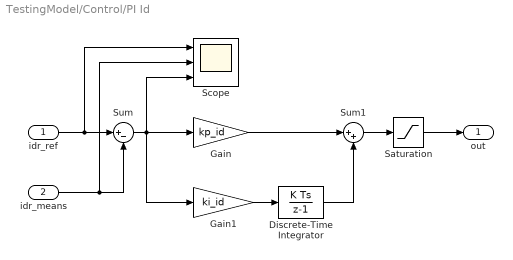
== system TestingModel/Control/PI Id ==
  idr_ref : Inport
  idr_means : Inport  Port=2
  Discrete-Time Integrator : DiscreteIntegrator  SampleTime=1/fsw  LimitOutput=on  UpperSaturationLimit=Vbus/sqrt(3)  LowerSaturationLimit=-Vbus/sqrt(3)  ICPrevOutput=DiscIntNeverNeededParam  ICPrevScaledInput=DiscIntNeverNeededParam
  Gain : Gain  Gain=kp_id
  Gain1 : Gain  Gain=ki_id
  Saturation : Saturate  UpperLimit=Vbus/sqrt(3)  LowerLimit=-Vbus/sqrt(3)
  Scope : Scope  NumInputPorts=3
  Sum : Sum  Inputs=|+-
  Sum1 : Sum  Inputs=|++
  out : Outport  VectorParamsAs1DForOutWhenUnconnected=off
  wires:
  idr_means/1 -> Scope/2, Sum/2
  idr_ref/1 -> Scope/1, Sum/1
  Sum/1 -> Scope/3, Gain1/1, Gain/1
  Gain/1 -> Sum1/1
  Gain1/1 -> Discrete-Time Integrator/1
  Discrete-Time Integrator/1 -> Sum1/2
  Sum1/1 -> Saturation/1
  Saturation/1 -> out/1

== system TestingModel/Control/PI Iq ==
  iqr_ref : Inport
  iqr_means : Inport  Port=2
  Discrete-Time Integrator : DiscreteIntegrator  SampleTime=1/fsw  LimitOutput=on  UpperSaturationLimit=Vbus/sqrt(3)  LowerSaturationLimit=-Vbus/sqrt(3)  ICPrevOutput=DiscIntNeverNeededParam  ICPrevScaledInput=DiscIntNeverNeededParam
  Gain : Gain  Gain=kp_iq
  Gain1 : Gain  Gain=ki_iq
  Saturation : Saturate  UpperLimit=Vbus/sqrt(3)  LowerLimit=-Vbus/sqrt(3)
  Sum : Sum  Inputs=|+-
  Sum1 : Sum  Inputs=|++
  out : Outport  VectorParamsAs1DForOutWhenUnconnected=off
  wires:
  iqr_means/1 -> Sum/2
  iqr_ref/1 -> Sum/1
  Sum/1 -> Gain1/1, Gain/1
  Gain/1 -> Sum1/1
  Gain1/1 -> Discrete-Time Integrator/1
  Discrete-Time Integrator/1 -> Sum1/2
  Sum1/1 -> Saturation/1
  Saturation/1 -> out/1

== system TestingModel/Control/abc -> DQ  ==
  note: iQr
  note: iDr
  iabcr : Inport
  Fcn : Fcn  Expr=2/3*(u[1]-u[2]/2-u[3]/2)
  Fcn1 : Fcn  Expr=2/3*(u[2]*(sqrt(3)/2)-u[3]*(sqrt(3)/2))
  Mux : Mux  Inputs=2
  i Dr/Qr : Outport  VectorParamsAs1DForOutWhenUnconnected=off
  wires:
  Mux/1 -> i Dr/Qr/1
  iabcr/1 -> Fcn1/1, Fcn/1
  Fcn/1 -> Mux/1
  Fcn1/1 -> Mux/2

== system TestingModel/Control/d//q -> D//Q  ==
  Vdr_ref  Vqr_ref : Inport
  theta_r (θr) : Inport  Port=2
  Fcn : Fcn  Expr=u(1)*cos(u[3])-u[2]*sin(u[3])
  Fcn1 : Fcn  Expr=u(1)*sin(u[3])+u[2]*cos(u[3])
  Mux : Mux  Inputs=2
  Mux1 : Mux  Inputs=2
  V Dr/Qr : Outport  VectorParamsAs1DForOutWhenUnconnected=off
  wires:
  Mux/1 -> V Dr/Qr/1
  Fcn/1 -> Mux/1
  Fcn1/1 -> Mux/2
  Vdr_ref  Vqr_ref/1 -> Mux1/1
  theta_r (θr)/1 -> Mux1/2
  Mux1/1 -> Fcn/1, Fcn1/1

== system TestingModel/Control/ Angle Rotor/Clarke: abc -> αβ  ==
  Vabc : Inport
  Fcn : Fcn  Expr=2/3*(u[1]-u[2]/2-u[3]/2)
  Fcn1 : Fcn  Expr=2/3*(u[2]*(sqrt(3)/2)-u[3]*(sqrt(3)/2))
  Mux : Mux  Inputs=2
  "Valfa/beta " : Outport  VectorParamsAs1DForOutWhenUnconnected=off
  wires:
  Mux/1 -> "Valfa/beta "/1
  Vabc/1 -> Fcn1/1, Fcn/1
  Fcn/1 -> Mux/1
  Fcn1/1 -> Mux/2
